simulink model "spaceShuttleOriginal"  (R2017b)
settings: Solver=FixedStepAuto  StartTime=0.0  StopTime=300  FixedStep=0.08  RelTol=1e-3
undefined symbols (not defined in the file or in its folder): ATTITUDE_ESTIMATE, ATTITUDE_INCREMENT, AUTO_MANUAL_SWITCH, BYPASS, COUNTER, CURRENT_ATTITUDE, DESIRED_ATTITUDE, DESIRED_RATE, INIT_AUTO_MANEUVER, INIT_JET_SELECT, INIT_STATE_ERROR, MANEUVER_HOLD_SW, PRIMARY_JET_COMMAND, RATE_ESTIMATE, UNDESIRED_ACCELERATION_ESTIMATE, VERNIER_JET_COMMAND
libraries: sharedtransform x5, aerolibutil x4, realtime_pacer_lib x1
(part 2 of 3)

== system spaceShuttleOriginal/State Error/Coordinate 2 ==
  In1 : Inport
  Bus Selector : BusSelector  OutputSignals=INIT_STATE_ERROR
  INIT STATE ERROR = OFF : Subsystem  TreatAsAtomicUnit=on
  INIT STATE ERROR = ON : Subsystem  TreatAsAtomicUnit=on
  If : If  IfExpression=u1 == 1
  Merge : Merge
  Selector : Selector  InputPortWidth=3  IndexOptions=Index vector (dialog)  Indices=[2]  OutputSizes=1
  y : Outport
  wires:
  Merge/1 -> y/1
  In1/1 -> INIT STATE ERROR = OFF/1(In1), INIT STATE ERROR = ON/1(In1), Bus Selector/1
  If/2 -> INIT STATE ERROR = OFF/Action
  INIT STATE ERROR = ON/1(y) -> Merge/1
  If/1 -> INIT STATE ERROR = ON/Action
  Selector/1 -> If/1
  INIT STATE ERROR = OFF/1(y1) -> Merge/2
  Bus Selector/1 -> Selector/1  "<INIT_STATE_ERROR>"

== system spaceShuttleOriginal/State Error/Coordinate 3 ==
  In2 : Inport
  Bus Selector : BusSelector  OutputSignals=INIT_STATE_ERROR
  INIT STATE ERROR = OFF : Subsystem  TreatAsAtomicUnit=on
  INIT STATE ERROR = ON : Subsystem  TreatAsAtomicUnit=on
  If : If  IfExpression=u1 == 1
  Merge : Merge
  Selector : Selector  InputPortWidth=3  IndexOptions=Index vector (dialog)  Indices=[3]  OutputSizes=1
  y1 : Outport
  wires:
  Merge/1 -> y1/1
  In2/1 -> INIT STATE ERROR = OFF/1(In1), INIT STATE ERROR = ON/1(In1), Bus Selector/1
  If/2 -> INIT STATE ERROR = OFF/Action
  INIT STATE ERROR = ON/1(y) -> Merge/1
  If/1 -> INIT STATE ERROR = ON/Action
  Selector/1 -> If/1
  INIT STATE ERROR = OFF/1(y1) -> Merge/2
  Bus Selector/1 -> Selector/1  "<INIT_STATE_ERROR>"

== system spaceShuttleOriginal/Update Auto Manual Switch/IF RHC ==
  In1 : Inport
  Action Port : ActionPort  ActionType=then
  Bus Assignment : BusAssignment  AssignedSignals=AUTO_MANUAL_SWITCH
  Constant1 : Constant  Value=0
  Data Store Read : DataStoreRead  DataStoreName=AUTO_MANUAL_SWITCH  DataStoreElements=AUTO_MANUAL_SWITCH(1)
  Data Store Write1 : DataStoreWrite  DataStoreName=AUTO_MANUAL_SWITCH
  Mux : Mux  Inputs=2
  x : Outport
  wires:
  Mux/1 -> Bus Assignment/2, Data Store Write1/1
  Data Store Read/1 -> Mux/2
  Constant1/1 -> Mux/1
  In1/1 -> Bus Assignment/1
  Bus Assignment/1 -> x/1

== system spaceShuttleOriginal/Update Auto Manual Switch/NO RHC ==
  In1 : Inport
  Action Port : ActionPort  ActionType=else
  Bus Assignment : BusAssignment  AssignedSignals=AUTO_MANUAL_SWITCH
  Constant1 : Constant
  Data Store Read : DataStoreRead  DataStoreName=AUTO_MANUAL_SWITCH  DataStoreElements=AUTO_MANUAL_SWITCH(1)
  Data Store Write1 : DataStoreWrite  DataStoreName=AUTO_MANUAL_SWITCH
  Mux : Mux  Inputs=2
  x1 : Outport
  wires:
  Mux/1 -> Bus Assignment/2, Data Store Write1/1
  Constant1/1 -> Mux/1
  Data Store Read/1 -> Mux/2
  Bus Assignment/1 -> x1/1
  In1/1 -> Bus Assignment/1

== system spaceShuttleOriginal/VISUALIZATION AND COMMANDS/Knob1 ==

== system spaceShuttleOriginal/VISUALIZATION AND COMMANDS/Knob2 ==

== system spaceShuttleOriginal/VISUALIZATION AND COMMANDS/Knob3 ==

== system spaceShuttleOriginal/VISUALIZATION AND COMMANDS/Knob4 ==

== system spaceShuttleOriginal/VISUALIZATION AND COMMANDS/Knob5 ==

== system spaceShuttleOriginal/VISUALIZATION AND COMMANDS/Lamp ==

== system spaceShuttleOriginal/VISUALIZATION AND COMMANDS/Lamp1 ==

== system spaceShuttleOriginal/VISUALIZATION AND COMMANDS/Lamp10 ==

== system spaceShuttleOriginal/VISUALIZATION AND COMMANDS/Lamp2 ==

== system spaceShuttleOriginal/VISUALIZATION AND COMMANDS/Lamp3 ==

== system spaceShuttleOriginal/VISUALIZATION AND COMMANDS/Lamp4 ==

== system spaceShuttleOriginal/VISUALIZATION AND COMMANDS/Lamp5 ==

== system spaceShuttleOriginal/VISUALIZATION AND COMMANDS/Lamp6 ==

== system spaceShuttleOriginal/VISUALIZATION AND COMMANDS/Lamp7 ==

== system spaceShuttleOriginal/VISUALIZATION AND COMMANDS/Lamp8 ==

== system spaceShuttleOriginal/VISUALIZATION AND COMMANDS/Lamp9 ==

== system spaceShuttleOriginal/VISUALIZATION AND COMMANDS/Rotary Switch ==

== system spaceShuttleOriginal/VISUALIZATION AND COMMANDS/Rotary Switch1 ==

== system spaceShuttleOriginal/VISUALIZATION AND COMMANDS/Rotary Switch2 ==

== system spaceShuttleOriginal/VISUALIZATION AND COMMANDS/Toggle Switch ==

== system spaceShuttleOriginal/VISUALIZATION AND COMMANDS/Toggle Switch1 ==

== system spaceShuttleOriginal/VISUALIZATION AND COMMANDS/Toggle Switch2 ==

== system spaceShuttleOriginal/VISUALIZATION AND COMMANDS/Toggle Switch3 ==

== system spaceShuttleOriginal/Attitude Processing/SECOND_PASS == 1/ATTITUDE PROCESSOR ==
  R_I_B : Inport
  R_I_B_PREVIOUS : Inport  Port=2
  Direction Cosine Matrix to Quaternions : sharedtransform/Direction Cosine Matrix  to Quaternions
      settings: SourceProductName=Aerospace Blockset  SourceProductBaseCode=AE
  Direction Cosine Matrix to Quaternions1 : sharedtransform/Direction Cosine Matrix  to Quaternions
      settings: SourceProductName=Aerospace Blockset  SourceProductBaseCode=AE
  Direction Cosine Matrix to Quaternions2 : sharedtransform/Direction Cosine Matrix  to Quaternions
      settings: SourceProductName=Aerospace Blockset  SourceProductBaseCode=AE
  Display1 : Display
  Display2 : Display
  Display3 : Display
  MATLAB Function2 : MATLAB Function  TreatAsAtomicUnit=on
  MATLAB Function3 : MATLAB Function  TreatAsAtomicUnit=on
  Quaternion Conjugate : aerolibutil/Quaternion Conjugate
      settings: SourceProductName=Aerospace Blockset  SourceProductBaseCode=AE
  Quaternion Multiplication : aerolibutil/Quaternion Multiplication
  Scope : Scope
  Scope1 : Scope
  To Workspace : ToWorkspace  VariableName=test1  SaveFormat=Timeseries  SampleTime=-1
  CURRENT ATTITUDE : Outport
  ATTITUDE INCREMENT : Outport  Port=2
  wires:
  R_I_B/1 -> Direction Cosine Matrix to Quaternions1/1, MATLAB Function3/1(u), Direction Cosine Matrix to Quaternions/1
  Direction Cosine Matrix to Quaternions/1 -> To Workspace/1, Scope/1, Display1/1, CURRENT ATTITUDE/1
  R_I_B_PREVIOUS/1 -> Direction Cosine Matrix to Quaternions2/1
  MATLAB Function2/1(x) -> Scope1/1, Display3/1, ATTITUDE INCREMENT/1
  MATLAB Function3/1(x) -> Display2/1
  Direction Cosine Matrix to Quaternions2/1 -> Quaternion Conjugate/1
  Direction Cosine Matrix to Quaternions1/1 -> Quaternion Multiplication/1
  Quaternion Conjugate/1 -> Quaternion Multiplication/2
  Quaternion Multiplication/1 -> MATLAB Function2/1(u)

== system spaceShuttleOriginal/Attitude Processing/SECOND_PASS == 1/State Estimator Part I ==
  CURRENT_ATTITUDE : Inport
  Derivative1 : Derivative
  Derivative2 : Derivative
  MATLAB Function2 : MATLAB Function  TreatAsAtomicUnit=on
  ATTITUDE_ESTIMATE : Outport
  RATE_ESTIMATE : Outport  Port=2
  UNDESIRED_ACCELERATION_ESTIMATE : Outport  Port=3
  wires:
  Derivative1/1 -> Derivative2/1, RATE_ESTIMATE/1
  Derivative2/1 -> UNDESIRED_ACCELERATION_ESTIMATE/1
  CURRENT_ATTITUDE/1 -> MATLAB Function2/1(u)
  MATLAB Function2/1(x) -> ATTITUDE_ESTIMATE/1, Derivative1/1

== system spaceShuttleOriginal/Auto // Manual Maneuver/IF MANUAL/MANUAL MANEUVER MODULE ==
  In1 : Inport
  Affect Coordinate 1 : Subsystem
  Affect Coordinate 2 : Subsystem
  Affect Coordinate 3 : Subsystem
  Out1 : Outport
  wires:
  In1/1 -> Affect Coordinate 1/1(In1)
  Affect Coordinate 1/1(Out1) -> Affect Coordinate 2/1(In1)
  Affect Coordinate 2/1(Out1) -> Affect Coordinate 3/1(In1)
  Affect Coordinate 3/1(Out1) -> Out1/1

== system spaceShuttleOriginal/Auto // Manual Maneuver/If AUTO/COUNTER ~=0 ==
  In1 : Inport
  Action Port : ActionPort  ActionType=else
  Out1 : Outport
  wires:
  In1/1 -> Out1/1

== system spaceShuttleOriginal/Auto // Manual Maneuver/If AUTO/IF COUNTER=0 ==
  In2 : Inport
  Action Port : ActionPort  ActionType=then
  AUTO MANEUVER MODULE : Subsystem
  Bus Assignment : BusAssignment  AssignedSignals=COUNTER
  Constant2 : Constant  Value=12
  Data Store Write1 : DataStoreWrite  DataStoreName=COUNTER
  Out1 : Outport
  wires:
  Constant2/1 -> Bus Assignment/2, Data Store Write1/1
  AUTO MANEUVER MODULE/1(Out1) -> Out1/1
  Bus Assignment/1 -> AUTO MANEUVER MODULE/1(In1)
  In2/1 -> Bus Assignment/1

== system spaceShuttleOriginal/Auto // Manual Maneuver/If AUTO/IF OLD=AUTO ==
  In1 : Inport
  Action Port : ActionPort  ActionType=else
  Out1 : Outport
  wires:
  In1/1 -> Out1/1

== system spaceShuttleOriginal/Auto // Manual Maneuver/If AUTO/IF OLD=MANUAL ==
  In1 : Inport
  Action Port : ActionPort  ActionType=then
  Bus Assignment : BusAssignment  AssignedSignals=BYPASS,INIT_AUTO_MANEUVER,COUNTER
  Constant{1..4} (4 alike) : Constant  Value=0
  Constant5 : Constant
  Data Store Write : DataStoreWrite  DataStoreName=BYPASS
  Data Store Write1 : DataStoreWrite  DataStoreName=COUNTER
  Data Store Write2 : DataStoreWrite  DataStoreName=INIT_AUTO_MANEUVER
  Mux : Mux  Inputs=3
  Out1 : Outport
  wires:
  Constant2/1 -> Bus Assignment/4, Data Store Write1/1
  Constant1/1 -> Mux/1
  Constant3/1 -> Mux/2
  Constant4/1 -> Mux/3
  Mux/1 -> Bus Assignment/2, Data Store Write/1
  Constant5/1 -> Bus Assignment/3, Data Store Write2/1
  In1/1 -> Bus Assignment/1
  Bus Assignment/1 -> Out1/1

== system spaceShuttleOriginal/First Pass/If First Pass/AUTO ==
  In2 : Inport
  Action Port : ActionPort  ActionType=else
  Bus Assignment1 : BusAssignment  AssignedSignals=INIT_STATE_ERROR
  Data Store Read : DataStoreRead  DataStoreName=INIT_STATE_ERROR
  x1 : Outport
  wires:
  Data Store Read/1 -> Bus Assignment1/2
  In2/1 -> Bus Assignment1/1
  Bus Assignment1/1 -> x1/1

== system spaceShuttleOriginal/First Pass/If First Pass/MANUAL ==
  In1 : Inport
  Action Port : ActionPort  ActionType=then
  Bus Assignment : BusAssignment  AssignedSignals=INIT_STATE_ERROR
  Constant2 : Constant  Value=[1;1;1]
  Data Store Write1 : DataStoreWrite  DataStoreName=INIT_STATE_ERROR
  x : Outport
  wires:
  In1/1 -> Bus Assignment/1
  Bus Assignment/1 -> x/1
  Constant2/1 -> Data Store Write1/1, Bus Assignment/2

== system spaceShuttleOriginal/State Error/Coordinate 1/INIT STATE ERROR = OFF ==
  In1 : Inport
  Action Port : ActionPort  ActionType=else
  y1 : Outport
  wires:
  In1/1 -> y1/1

== system spaceShuttleOriginal/State Error/Coordinate 1/INIT STATE ERROR = ON ==
  In1 : Inport
  Action Port : ActionPort  ActionType=then
  Bus Assignment : BusAssignment  AssignedSignals=DESIRED_ATTITUDE
  Bus Assignment1 : BusAssignment  AssignedSignals=INIT_STATE_ERROR
  Bus Selector : BusSelector  OutputSignals=DESIRED_ATTITUDE,ATTITUDE_ESTIMATE
  Bus Selector1 : BusSelector  OutputSignals=INIT_STATE_ERROR
  Constant : Constant  Value=0
  Data Store Write1 : DataStoreWrite  DataStoreName=INIT_STATE_ERROR
  Data Store Write3 : DataStoreWrite  DataStoreName=DESIRED_ATTITUDE
  Demux : Demux  Outputs=3
  Demux1 : Demux  Outputs=3
  Mux : Mux  Inputs=3
  Mux1 : Mux  Inputs=3
  Selector : Selector  InputPortWidth=3  IndexOptions=Index vector (dialog)  Indices=[1]  OutputSizes=1
  Terminator : Terminator
  Terminator1 : Terminator
  y : Outport
  wires:
  In1/1 -> Bus Assignment/1, Bus Selector/1
  Bus Selector/1 -> Demux/1  "<DESIRED_ATTITUDE>"
  Bus Selector/2 -> Selector/1  "<ATTITUDE_ESTIMATE>"
  Selector/1 -> Mux/1
  Demux/2 -> Mux/2
  Demux/3 -> Mux/3
  Mux/1 -> Data Store Write3/1, Bus Assignment/2
  Bus Selector1/1 -> Demux1/1  "<INIT_STATE_ERROR>"
  Demux1/3 -> Mux1/3
  Bus Assignment1/1 -> y/1
  Mux1/1 -> Bus Assignment1/2, Data Store Write1/1
  Bus Assignment/1 -> Bus Assignment1/1, Bus Selector1/1
  Demux1/2 -> Mux1/2
  Constant/1 -> Mux1/1
  Demux/1 -> Terminator/1
  Demux1/1 -> Terminator1/1

== system spaceShuttleOriginal/State Error/Coordinate 2/INIT STATE ERROR = OFF ==
  In1 : Inport
  Action Port : ActionPort  ActionType=else
  y1 : Outport
  wires:
  In1/1 -> y1/1

== system spaceShuttleOriginal/State Error/Coordinate 2/INIT STATE ERROR = ON ==
  In1 : Inport
  Action Port : ActionPort  ActionType=then
  Bus Assignment : BusAssignment  AssignedSignals=DESIRED_ATTITUDE
  Bus Assignment1 : BusAssignment  AssignedSignals=INIT_STATE_ERROR
  Bus Selector : BusSelector  OutputSignals=DESIRED_ATTITUDE,ATTITUDE_ESTIMATE
  Bus Selector1 : BusSelector  OutputSignals=INIT_STATE_ERROR
  Constant : Constant  Value=0
  Data Store Write1 : DataStoreWrite  DataStoreName=INIT_STATE_ERROR
  Data Store Write3 : DataStoreWrite  DataStoreName=DESIRED_ATTITUDE
  Demux : Demux  Outputs=3
  Demux1 : Demux  Outputs=3
  Mux : Mux  Inputs=3
  Mux1 : Mux  Inputs=3
  Selector : Selector  InputPortWidth=3  IndexOptions=Index vector (dialog)  Indices=[2]  OutputSizes=1
  Terminator : Terminator
  Terminator1 : Terminator
  y : Outport
  wires:
  In1/1 -> Bus Assignment/1, Bus Selector/1
  Bus Selector/1 -> Demux/1  "<DESIRED_ATTITUDE>"
  Bus Selector/2 -> Selector/1  "<ATTITUDE_ESTIMATE>"
  Mux/1 -> Data Store Write3/1, Bus Assignment/2
  Bus Selector1/1 -> Demux1/1  "<INIT_STATE_ERROR>"
  Bus Assignment1/1 -> y/1
  Mux1/1 -> Bus Assignment1/2, Data Store Write1/1
  Bus Assignment/1 -> Bus Assignment1/1, Bus Selector1/1
  Selector/1 -> Mux/2
  Demux/3 -> Mux/3
  Demux/1 -> Mux/1
  Constant/1 -> Mux1/2
  Demux1/1 -> Mux1/1
  Demux1/3 -> Mux1/3
  Demux/2 -> Terminator/1
  Demux1/2 -> Terminator1/1

== system spaceShuttleOriginal/State Error/Coordinate 3/INIT STATE ERROR = OFF ==
  In1 : Inport
  Action Port : ActionPort  ActionType=else
  y1 : Outport
  wires:
  In1/1 -> y1/1

== system spaceShuttleOriginal/State Error/Coordinate 3/INIT STATE ERROR = ON ==
  In1 : Inport
  Action Port : ActionPort  ActionType=then
  Bus Assignment : BusAssignment  AssignedSignals=DESIRED_ATTITUDE
  Bus Assignment1 : BusAssignment  AssignedSignals=INIT_STATE_ERROR
  Bus Selector : BusSelector  OutputSignals=DESIRED_ATTITUDE,ATTITUDE_ESTIMATE
  Bus Selector1 : BusSelector  OutputSignals=INIT_STATE_ERROR
  Constant : Constant  Value=0
  Data Store Write1 : DataStoreWrite  DataStoreName=INIT_STATE_ERROR
  Data Store Write3 : DataStoreWrite  DataStoreName=DESIRED_ATTITUDE
  Demux : Demux  Outputs=3
  Demux1 : Demux  Outputs=3
  Mux : Mux  Inputs=3
  Mux1 : Mux  Inputs=3
  Selector : Selector  InputPortWidth=3  IndexOptions=Index vector (dialog)  Indices=[3]  OutputSizes=1
  Terminator : Terminator
  Terminator1 : Terminator
  y : Outport
  wires:
  In1/1 -> Bus Assignment/1, Bus Selector/1
  Bus Selector/1 -> Demux/1  "<DESIRED_ATTITUDE>"
  Bus Selector/2 -> Selector/1  "<ATTITUDE_ESTIMATE>"
  Mux/1 -> Data Store Write3/1, Bus Assignment/2
  Bus Selector1/1 -> Demux1/1  "<INIT_STATE_ERROR>"
  Bus Assignment1/1 -> y/1
  Mux1/1 -> Bus Assignment1/2, Data Store Write1/1
  Bus Assignment/1 -> Bus Assignment1/1, Bus Selector1/1
  Selector/1 -> Mux/3
  Demux/2 -> Mux/2
  Demux/1 -> Mux/1
  Constant/1 -> Mux1/3
  Demux1/2 -> Mux1/2
  Demux1/1 -> Mux1/1
  Demux/3 -> Terminator/1
  Demux1/3 -> Terminator1/1

== system spaceShuttleOriginal/Auto // Manual Maneuver/IF MANUAL/MANUAL MANEUVER MODULE/Affect Coordinate 1 ==
  In1 : Inport
  Bus Selector : BusSelector  OutputSignals=USER_INPUTS.CLOSED_LOOP
  CLOSED LOOP = OFF : Subsystem  TreatAsAtomicUnit=on
  CLOSED LOOP = ON : Subsystem  TreatAsAtomicUnit=on
  If : If  IfExpression=u1 == 1
  Merge : Merge
  Selector : Selector  InputPortWidth=3  IndexOptions=Index vector (dialog)  Indices=[1]  OutputSizes=1
  Out1 : Outport
  wires:
  In1/1 -> CLOSED LOOP = ON/1(x), CLOSED LOOP = OFF/1(x), Bus Selector/1
  Bus Selector/1 -> Selector/1  "<CLOSED_LOOP>"
  Merge/1 -> Out1/1
  CLOSED LOOP = OFF/1(y) -> Merge/2
  Selector/1 -> If/1
  If/2 -> CLOSED LOOP = OFF/Action
  If/1 -> CLOSED LOOP = ON/Action
  CLOSED LOOP = ON/1(Out2) -> Merge/1

== system spaceShuttleOriginal/Auto // Manual Maneuver/IF MANUAL/MANUAL MANEUVER MODULE/Affect Coordinate 2 ==
  In1 : Inport
  Bus Selector : BusSelector  OutputSignals=USER_INPUTS.CLOSED_LOOP
  CLOSED LOOP = OFF : Subsystem  TreatAsAtomicUnit=on
  CLOSED LOOP = ON : Subsystem  TreatAsAtomicUnit=on
  If : If  IfExpression=u1 == 1
  Merge : Merge
  Selector : Selector  InputPortWidth=3  IndexOptions=Index vector (dialog)  Indices=[2]  OutputSizes=1
  Out1 : Outport
  wires:
  In1/1 -> CLOSED LOOP = OFF/1(x), CLOSED LOOP = ON/1(x), Bus Selector/1
  Bus Selector/1 -> Selector/1  "<CLOSED_LOOP>"
  Merge/1 -> Out1/1
  CLOSED LOOP = OFF/1(y) -> Merge/2
  Selector/1 -> If/1
  If/2 -> CLOSED LOOP = OFF/Action
  If/1 -> CLOSED LOOP = ON/Action
  CLOSED LOOP = ON/1(Out1) -> Merge/1

== system spaceShuttleOriginal/Auto // Manual Maneuver/IF MANUAL/MANUAL MANEUVER MODULE/Affect Coordinate 3 ==
  In1 : Inport
  Bus Selector : BusSelector  OutputSignals=USER_INPUTS.CLOSED_LOOP
  CLOSED LOOP = OFF : Subsystem  TreatAsAtomicUnit=on
  CLOSED LOOP = ON : Subsystem  TreatAsAtomicUnit=on
  If : If  IfExpression=u1 == 1
  Merge : Merge
  Selector : Selector  InputPortWidth=3  IndexOptions=Index vector (dialog)  Indices=[3]  OutputSizes=1
  Out1 : Outport
  wires:
  In1/1 -> CLOSED LOOP = ON/1(x), CLOSED LOOP = OFF/1(x), Bus Selector/1
  Bus Selector/1 -> Selector/1  "<CLOSED_LOOP>"
  Merge/1 -> Out1/1
  CLOSED LOOP = OFF/1(y) -> Merge/2
  Selector/1 -> If/1
  If/2 -> CLOSED LOOP = OFF/Action
  If/1 -> CLOSED LOOP = ON/Action
  CLOSED LOOP = ON/1(Out1) -> Merge/1

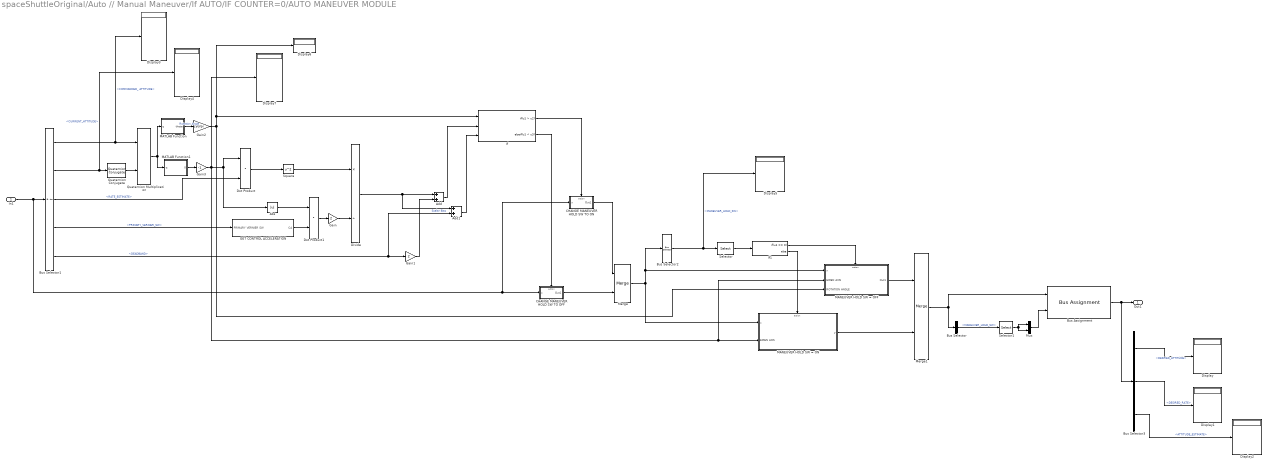
== system spaceShuttleOriginal/Auto // Manual Maneuver/If AUTO/IF COUNTER=0/AUTO MANEUVER MODULE ==
  In1 : Inport
  Abs : Abs
  Add : Sum
  Add1 : Sum
  Bus Assignment : BusAssignment  AssignedSignals=MANEUVER_HOLD_SW
  Bus Selector : BusSelector  OutputSignals=MANEUVER_HOLD_SW
  Bus Selector1 : BusSelector  OutputSignals=USER_INPUTS.COMMANDED_ ATTITUDE,CURRENT_ATTITUDE,RATE_ESTIMATE,USER_INPUTS.PRIMARY_VERNIER_SW,USER_INPUTS.DEADBAND
  Bus Selector2 : BusSelector  OutputSignals=MANEUVER_HOLD_SW
  Bus Selector3 : BusSelector  OutputSignals=DESIRED_ATTITUDE,DESIRED_RATE,ATTITUDE_ESTIMATE
  CHANGE MANEUVER HOLD SW TO OFF : Subsystem  TreatAsAtomicUnit=on
  CHANGE MANEUVER HOLD SW TO ON : Subsystem  TreatAsAtomicUnit=on
  Display{,1..7} (8 alike) : Display
  Divide : Product  Inputs=*/
  Dot Product : DotProduct  InputSameDT=on  OutDataTypeStr=Inherit: Inherit via internal rule
  Dot Product1 : DotProduct  InputSameDT=on  OutDataTypeStr=Inherit: Inherit via internal rule
  GET CONTROL ACCELERATION : Subsystem
  Gain : Gain  Gain=2
  Gain1 : Gain  Gain=2
  Gain2 : Gain  Gain=180/pi
  Gain3 : Gain  Gain=-1
  If : If  NumInputs=3  IfExpression=u1 > u2  ElseIfExpressions=u1 < u3  ShowElse=off
  If1 : If  IfExpression=u1 == 0
  MANEUVER HOLD SW = OFF : Subsystem  TreatAsAtomicUnit=on
  MANEUVER HOLD SW = ON : Subsystem  TreatAsAtomicUnit=on
  MATLAB Function : MATLAB Function  TreatAsAtomicUnit=on
  MATLAB Function1 : MATLAB Function  TreatAsAtomicUnit=on
  Merge : Merge
  Merge1 : Merge
  Mux : Mux  Inputs=2
  Quaternion Conjugate : aerolibutil/Quaternion Conjugate
      settings: SourceProductName=Aerospace Blockset  SourceProductBaseCode=AE
  Quaternion Multiplication : aerolibutil/Quaternion Multiplication
  Selector : Selector  InputPortWidth=2  IndexOptions=Index vector (dialog)  Indices=[1]  OutputSizes=1
  Selector1 : Selector  InputPortWidth=2  IndexOptions=Index vector (dialog)  Indices=[1]  OutputSizes=1
  Square : Math  Operator=square  RndMeth=Zero  SaturateOnIntegerOverflow=on
  Out1 : Outport
  wires:
  MANEUVER HOLD SW = ON/1(y) -> Merge1/2
  Gain/1 -> Divide/2
  Divide/1 -> Add1/1, Add/1  "Scalar Bias"
  Merge/1 -> MANEUVER HOLD SW = ON/1(x), Bus Selector2/1, MANEUVER HOLD SW = OFF/1(x)
  If1/1 -> MANEUVER HOLD SW = OFF/Action
  CHANGE MANEUVER HOLD SW TO OFF/1(Out1) -> Merge/2
  MANEUVER HOLD SW = OFF/1(Out1) -> Merge1/1
  Selector/1 -> If1/1
  MATLAB Function1/1(U) -> Gain3/1
  Gain1/1 -> Add/2
  Add/1 -> If/2
  In1/1 -> Bus Selector1/1, CHANGE MANEUVER HOLD SW TO OFF/1(x), CHANGE MANEUVER HOLD SW TO ON/1(x)
  GET CONTROL ACCELERATION/1(CA) -> Dot Product1/2
  If/1 -> CHANGE MANEUVER HOLD SW TO ON/Action
  Square/1 -> Divide/1
  Dot Product1/1 -> Gain/1
  Add1/1 -> If/3
  MATLAB Function/1(theta) -> Gain2/1  "Rotation Angle"
  If/2 -> CHANGE MANEUVER HOLD SW TO OFF/Action
  Abs/1 -> Dot Product1/1
  Quaternion Multiplication/1 -> MATLAB Function/1(q), MATLAB Function1/1(q)
  If1/2 -> MANEUVER HOLD SW = ON/Action
  Quaternion Conjugate/1 -> Quaternion Multiplication/2
  Dot Product/1 -> Square/1
  CHANGE MANEUVER HOLD SW TO ON/1(Out1) -> Merge/1
  Bus Selector2/1 -> Display5/1, Selector/1  "<MANEUVER_HOLD_SW>"
  Merge1/1 -> Bus Selector/1, Bus Assignment/1
  Bus Selector/1 -> Selector1/1  "<MANEUVER_HOLD_SW>"
  Mux/1 -> Bus Assignment/2
  Selector1/1 -> Mux/1, Mux/2
  Bus Selector3/2 -> Display1/1  "<DESIRED_RATE>"
  Bus Selector3/1 -> Display/1  "<DESIRED_ATTITUDE>"
  Bus Assignment/1 -> Bus Selector3/1, Out1/1
  Bus Selector3/3 -> Display2/1  "<ATTITUDE_ESTIMATE>"
  Gain2/1 -> MANEUVER HOLD SW = OFF/3(ROTATION ANGLE), Display6/1, If/1
  Gain3/1 -> Display7/1, MANEUVER HOLD SW = OFF/2(EIGEN AXIS), MANEUVER HOLD SW = ON/2(EIGEN AXIS), Abs/1, Dot Product/1
  Bus Selector1/2 -> Quaternion Conjugate/1, Display4/1  "<CURRENT_ATTITUDE>"
  Bus Selector1/3 -> Dot Product/2  "<RATE_ESTIMATE>"
  Bus Selector1/4 -> GET CONTROL ACCELERATION/1(PRIMARY VERNIER SW)  "<PRIMARY_VERNIER_SW>"
  Bus Selector1/5 -> Add1/2, Gain1/1  "<DEADBAND>"
  Bus Selector1/1 -> Quaternion Multiplication/1, Display3/1  "<COMMANDED_ ATTITUDE>"

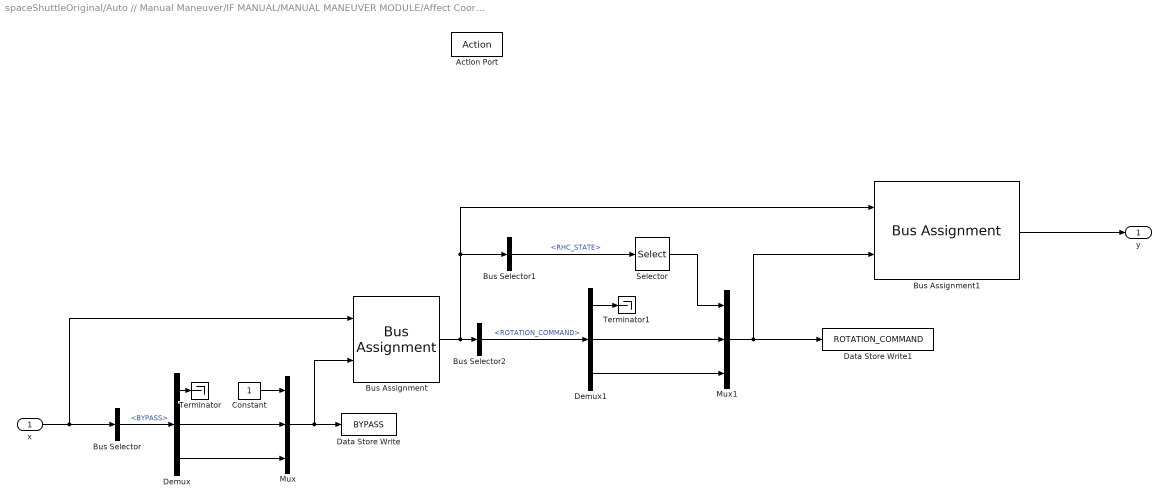
== system spaceShuttleOriginal/Auto // Manual Maneuver/IF MANUAL/MANUAL MANEUVER MODULE/Affect Coordinate 1/CLOSED LOOP = OFF ==
  x : Inport
  Action Port : ActionPort  ActionType=else
  Bus Assignment : BusAssignment  AssignedSignals=BYPASS
  Bus Assignment1 : BusAssignment  AssignedSignals=ROTATION_COMMAND
  Bus Selector : BusSelector  OutputSignals=BYPASS
  Bus Selector1 : BusSelector  OutputSignals=USER_INPUTS.RHC_STATE
  Bus Selector2 : BusSelector  OutputSignals=ROTATION_COMMAND
  Constant : Constant
  Data Store Write : DataStoreWrite  DataStoreName=BYPASS
  Data Store Write1 : DataStoreWrite  DataStoreName=ROTATION_COMMAND
  Demux : Demux  Outputs=3
  Demux1 : Demux  Outputs=3
  Mux : Mux  Inputs=3
  Mux1 : Mux  Inputs=3
  Selector : Selector  InputPortWidth=3  IndexOptions=Index vector (dialog)  Indices=[1]  OutputSizes=1
  Terminator : Terminator
  Terminator1 : Terminator
  y : Outport
  wires:
  x/1 -> Bus Assignment/1, Bus Selector/1
  Bus Selector/1 -> Demux/1  "<BYPASS>"
  Demux/3 -> Mux/3
  Demux/2 -> Mux/2
  Constant/1 -> Mux/1
  Mux/1 -> Data Store Write/1, Bus Assignment/2
  Demux/1 -> Terminator/1
  Bus Assignment/1 -> Bus Assignment1/1, Bus Selector1/1, Bus Selector2/1
  Mux1/1 -> Data Store Write1/1, Bus Assignment1/2
  Demux1/2 -> Mux1/2
  Demux1/3 -> Mux1/3
  Bus Selector2/1 -> Demux1/1  "<ROTATION_COMMAND>"
  Demux1/1 -> Terminator1/1
  Bus Selector1/1 -> Selector/1  "<RHC_STATE>"
  Selector/1 -> Mux1/1
  Bus Assignment1/1 -> y/1

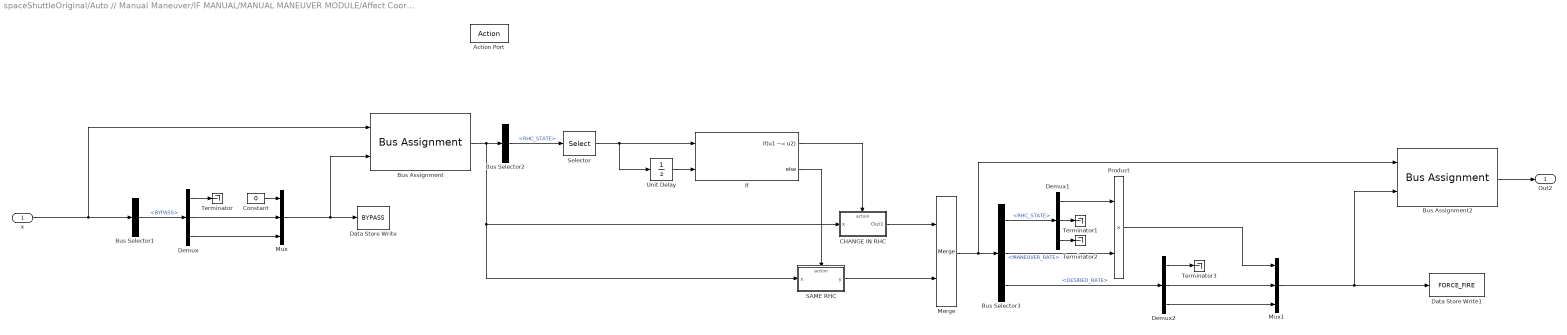
== system spaceShuttleOriginal/Auto // Manual Maneuver/IF MANUAL/MANUAL MANEUVER MODULE/Affect Coordinate 1/CLOSED LOOP = ON ==
  x : Inport
  Action Port : ActionPort  ActionType=then
  Bus Assignment : BusAssignment  AssignedSignals=BYPASS
  Bus Assignment2 : BusAssignment  AssignedSignals=FORCE_FIRE
  Bus Selector1 : BusSelector  OutputSignals=BYPASS
  Bus Selector2 : BusSelector  OutputSignals=USER_INPUTS.RHC_STATE
  Bus Selector3 : BusSelector  OutputSignals=USER_INPUTS.RHC_STATE,USER_INPUTS.MANEUVER_RATE,DESIRED_RATE
  CHANGE IN RHC : Subsystem  TreatAsAtomicUnit=on
  Constant : Constant  Value=0
  Data Store Write : DataStoreWrite  DataStoreName=BYPASS
  Data Store Write1 : DataStoreWrite  DataStoreName=FORCE_FIRE
  Demux : Demux  Outputs=3
  Demux1 : Demux  Outputs=3
  Demux2 : Demux  Outputs=3
  If : If  NumInputs=2  IfExpression=u1 ~= u2
  Merge : Merge
  Mux : Mux  Inputs=3
  Mux1 : Mux  Inputs=3
  Product : Product
  SAME RHC : Subsystem  TreatAsAtomicUnit=on
  Selector : Selector  InputPortWidth=3  IndexOptions=Index vector (dialog)  Indices=[1]  OutputSizes=1
  Terminator{,1..3} (4 alike) : Terminator
  Unit Delay : UnitDelay  SampleTime=-1
  Out2 : Outport
  wires:
  x/1 -> Bus Assignment/1, Bus Selector1/1
  Bus Selector1/1 -> Demux/1  "<BYPASS>"
  Constant/1 -> Mux/1
  Demux/2 -> Mux/2
  Demux/3 -> Mux/3
  Mux/1 -> Data Store Write/1, Bus Assignment/2
  Bus Assignment/1 -> CHANGE IN RHC/1(x), SAME RHC/1(x), Bus Selector2/1
  Bus Selector2/1 -> Selector/1  "<RHC_STATE>"
  Selector/1 -> Unit Delay/1, If/1
  Unit Delay/1 -> If/2
  SAME RHC/1(y) -> Merge/2
  If/2 -> SAME RHC/Action
  If/1 -> CHANGE IN RHC/Action
  CHANGE IN RHC/1(Out1) -> Merge/1
  Merge/1 -> Bus Assignment2/1, Bus Selector3/1
  Bus Selector3/1 -> Demux1/1  "<RHC_STATE>"
  Bus Assignment2/1 -> Out2/1
  Demux1/1 -> Product/1
  Bus Selector3/2 -> Product/2  "<MANEUVER_RATE>"
  Product/1 -> Mux1/1
  Bus Selector3/3 -> Demux2/1  "<DESIRED_RATE>"
  Demux2/3 -> Mux1/3
  Demux2/2 -> Mux1/2
  Mux1/1 -> Bus Assignment2/2, Data Store Write1/1
  Demux/1 -> Terminator/1
  Demux1/2 -> Terminator1/1
  Demux1/3 -> Terminator2/1
  Demux2/1 -> Terminator3/1

== system spaceShuttleOriginal/Auto // Manual Maneuver/IF MANUAL/MANUAL MANEUVER MODULE/Affect Coordinate 2/CLOSED LOOP = OFF ==
  x : Inport
  Action Port : ActionPort  ActionType=else
  Bus Assignment : BusAssignment  AssignedSignals=BYPASS
  Bus Assignment1 : BusAssignment  AssignedSignals=ROTATION_COMMAND
  Bus Selector : BusSelector  OutputSignals=BYPASS
  Bus Selector1 : BusSelector  OutputSignals=USER_INPUTS.RHC_STATE
  Bus Selector2 : BusSelector  OutputSignals=ROTATION_COMMAND
  Constant : Constant
  Data Store Write : DataStoreWrite  DataStoreName=BYPASS
  Data Store Write1 : DataStoreWrite  DataStoreName=ROTATION_COMMAND
  Demux : Demux  Outputs=3
  Demux1 : Demux  Outputs=3
  Mux : Mux  Inputs=3
  Mux1 : Mux  Inputs=3
  Selector : Selector  InputPortWidth=3  IndexOptions=Index vector (dialog)  Indices=[2]  OutputSizes=1
  Terminator : Terminator
  Terminator1 : Terminator
  y : Outport
  wires:
  x/1 -> Bus Assignment/1, Bus Selector/1
  Bus Selector/1 -> Demux/1  "<BYPASS>"
  Mux/1 -> Data Store Write/1, Bus Assignment/2
  Bus Assignment/1 -> Bus Assignment1/1, Bus Selector1/1, Bus Selector2/1
  Mux1/1 -> Data Store Write1/1, Bus Assignment1/2
  Bus Selector2/1 -> Demux1/1  "<ROTATION_COMMAND>"
  Bus Selector1/1 -> Selector/1  "<RHC_STATE>"
  Bus Assignment1/1 -> y/1
  Demux1/2 -> Terminator1/1
  Selector/1 -> Mux1/2
  Demux1/1 -> Mux1/1
  Demux1/3 -> Mux1/3
  Constant/1 -> Mux/2
  Demux/2 -> Terminator/1
  Demux/1 -> Mux/1
  Demux/3 -> Mux/3

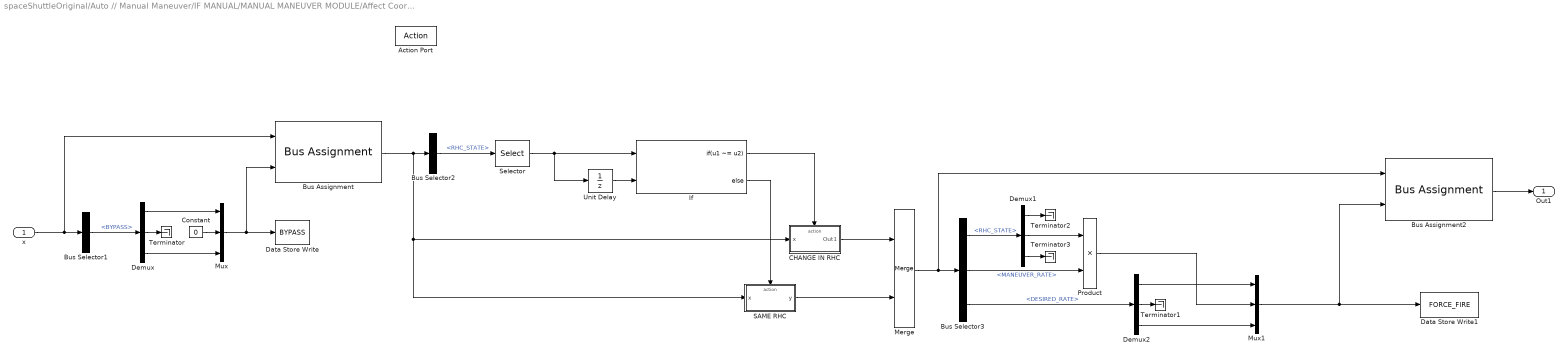
== system spaceShuttleOriginal/Auto // Manual Maneuver/IF MANUAL/MANUAL MANEUVER MODULE/Affect Coordinate 2/CLOSED LOOP = ON ==
  x : Inport
  Action Port : ActionPort  ActionType=then
  Bus Assignment : BusAssignment  AssignedSignals=BYPASS
  Bus Assignment2 : BusAssignment  AssignedSignals=FORCE_FIRE
  Bus Selector1 : BusSelector  OutputSignals=BYPASS
  Bus Selector2 : BusSelector  OutputSignals=USER_INPUTS.RHC_STATE
  Bus Selector3 : BusSelector  OutputSignals=USER_INPUTS.RHC_STATE,USER_INPUTS.MANEUVER_RATE,DESIRED_RATE
  CHANGE IN RHC : Subsystem  TreatAsAtomicUnit=on
  Constant : Constant  Value=0
  Data Store Write : DataStoreWrite  DataStoreName=BYPASS
  Data Store Write1 : DataStoreWrite  DataStoreName=FORCE_FIRE
  Demux : Demux  Outputs=3
  Demux1 : Demux  Outputs=3
  Demux2 : Demux  Outputs=3
  If : If  NumInputs=2  IfExpression=u1 ~= u2
  Merge : Merge
  Mux : Mux  Inputs=3
  Mux1 : Mux  Inputs=3
  Product : Product
  SAME RHC : Subsystem  TreatAsAtomicUnit=on
  Selector : Selector  InputPortWidth=3  IndexOptions=Index vector (dialog)  Indices=[2]  OutputSizes=1
  Terminator{,1..3} (4 alike) : Terminator
  Unit Delay : UnitDelay  SampleTime=-1
  Out1 : Outport
  wires:
  x/1 -> Bus Assignment/1, Bus Selector1/1
  Bus Selector1/1 -> Demux/1  "<BYPASS>"
  Demux/3 -> Mux/3
  Mux/1 -> Data Store Write/1, Bus Assignment/2
  Bus Assignment/1 -> CHANGE IN RHC/1(x), SAME RHC/1(x), Bus Selector2/1
  Bus Selector2/1 -> Selector/1  "<RHC_STATE>"
  Selector/1 -> Unit Delay/1, If/1
  Unit Delay/1 -> If/2
  SAME RHC/1(y) -> Merge/2
  If/2 -> SAME RHC/Action
  If/1 -> CHANGE IN RHC/Action
  CHANGE IN RHC/1(Out1) -> Merge/1
  Constant/1 -> Mux/2
  Demux/1 -> Mux/1
  Mux1/1 -> Bus Assignment2/2, Data Store Write1/1
  Demux2/3 -> Mux1/3
  Bus Selector3/2 -> Product/2  "<MANEUVER_RATE>"
  Bus Selector3/1 -> Demux1/1  "<RHC_STATE>"
  Bus Selector3/3 -> Demux2/1  "<DESIRED_RATE>"
  Bus Assignment2/1 -> Out1/1
  Merge/1 -> Bus Assignment2/1, Bus Selector3/1
  Demux1/2 -> Product/1
  Product/1 -> Mux1/2
  Demux2/1 -> Mux1/1
  Demux/2 -> Terminator/1
  Demux2/2 -> Terminator1/1
  Demux1/1 -> Terminator2/1
  Demux1/3 -> Terminator3/1

== system spaceShuttleOriginal/Auto // Manual Maneuver/IF MANUAL/MANUAL MANEUVER MODULE/Affect Coordinate 3/CLOSED LOOP = OFF ==
  x : Inport
  Action Port : ActionPort  ActionType=else
  Bus Assignment : BusAssignment  AssignedSignals=BYPASS
  Bus Assignment1 : BusAssignment  AssignedSignals=ROTATION_COMMAND
  Bus Selector : BusSelector  OutputSignals=BYPASS
  Bus Selector1 : BusSelector  OutputSignals=USER_INPUTS.RHC_STATE
  Bus Selector2 : BusSelector  OutputSignals=ROTATION_COMMAND
  Constant : Constant
  Data Store Write : DataStoreWrite  DataStoreName=BYPASS
  Data Store Write1 : DataStoreWrite  DataStoreName=ROTATION_COMMAND
  Demux : Demux  Outputs=3
  Demux1 : Demux  Outputs=3
  Mux : Mux  Inputs=3
  Mux1 : Mux  Inputs=3
  Selector : Selector  InputPortWidth=3  IndexOptions=Index vector (dialog)  Indices=[3]  OutputSizes=1
  Terminator : Terminator
  Terminator1 : Terminator
  y : Outport
  wires:
  x/1 -> Bus Assignment/1, Bus Selector/1
  Bus Selector/1 -> Demux/1  "<BYPASS>"
  Mux/1 -> Data Store Write/1, Bus Assignment/2
  Demux/1 -> Mux/1
  Bus Assignment/1 -> Bus Assignment1/1, Bus Selector1/1, Bus Selector2/1
  Mux1/1 -> Data Store Write1/1, Bus Assignment1/2
  Bus Selector2/1 -> Demux1/1  "<ROTATION_COMMAND>"
  Bus Selector1/1 -> Selector/1  "<RHC_STATE>"
  Bus Assignment1/1 -> y/1
  Constant/1 -> Mux/3
  Demux/3 -> Terminator/1
  Demux/2 -> Mux/2
  Demux1/3 -> Terminator1/1
  Demux1/1 -> Mux1/1
  Demux1/2 -> Mux1/2
  Selector/1 -> Mux1/3

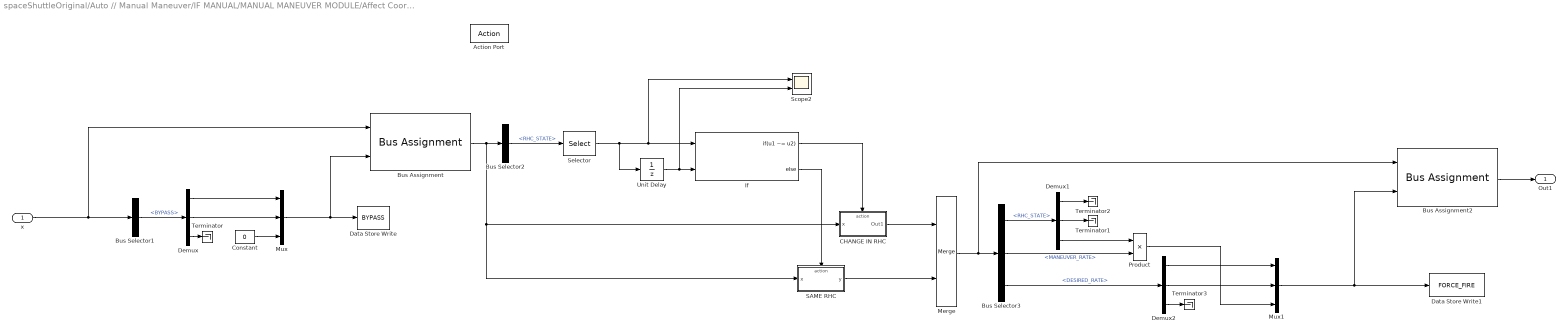
== system spaceShuttleOriginal/Auto // Manual Maneuver/IF MANUAL/MANUAL MANEUVER MODULE/Affect Coordinate 3/CLOSED LOOP = ON ==
  x : Inport
  Action Port : ActionPort  ActionType=then
  Bus Assignment : BusAssignment  AssignedSignals=BYPASS
  Bus Assignment2 : BusAssignment  AssignedSignals=FORCE_FIRE
  Bus Selector1 : BusSelector  OutputSignals=BYPASS
  Bus Selector2 : BusSelector  OutputSignals=USER_INPUTS.RHC_STATE
  Bus Selector3 : BusSelector  OutputSignals=USER_INPUTS.RHC_STATE,USER_INPUTS.MANEUVER_RATE,DESIRED_RATE
  CHANGE IN RHC : Subsystem  TreatAsAtomicUnit=on
  Constant : Constant  Value=0
  Data Store Write : DataStoreWrite  DataStoreName=BYPASS
  Data Store Write1 : DataStoreWrite  DataStoreName=FORCE_FIRE
  Demux : Demux  Outputs=3
  Demux1 : Demux  Outputs=3
  Demux2 : Demux  Outputs=3
  If : If  NumInputs=2  IfExpression=u1 ~= u2
  Merge : Merge
  Mux : Mux  Inputs=3
  Mux1 : Mux  Inputs=3
  Product : Product
  SAME RHC : Subsystem  TreatAsAtomicUnit=on
  Scope2 : Scope  NumInputPorts=2
  Selector : Selector  InputPortWidth=3  IndexOptions=Index vector (dialog)  Indices=[3]  OutputSizes=1
  Terminator{,1..3} (4 alike) : Terminator
  Unit Delay : UnitDelay  SampleTime=-1
  Out1 : Outport
  wires:
  x/1 -> Bus Assignment/1, Bus Selector1/1
  Bus Selector1/1 -> Demux/1  "<BYPASS>"
  Mux/1 -> Data Store Write/1, Bus Assignment/2
  Bus Assignment/1 -> CHANGE IN RHC/1(x), SAME RHC/1(x), Bus Selector2/1
  Bus Selector2/1 -> Selector/1  "<RHC_STATE>"
  Selector/1 -> Unit Delay/1, Scope2/1, If/1
  Unit Delay/1 -> Scope2/2, If/2
  SAME RHC/1(y) -> Merge/2
  If/2 -> SAME RHC/Action
  If/1 -> CHANGE IN RHC/Action
  CHANGE IN RHC/1(Out1) -> Merge/1
  Constant/1 -> Mux/3
  Demux/2 -> Mux/2
  Demux/1 -> Mux/1
  Bus Selector3/3 -> Demux2/1  "<DESIRED_RATE>"
  Bus Assignment2/1 -> Out1/1
  Bus Selector3/2 -> Product/2  "<MANEUVER_RATE>"
  Bus Selector3/1 -> Demux1/1  "<RHC_STATE>"
  Merge/1 -> Bus Assignment2/1, Bus Selector3/1
  Mux1/1 -> Bus Assignment2/2, Data Store Write1/1
  Demux1/3 -> Product/1
  Product/1 -> Mux1/3
  Demux2/1 -> Mux1/1
  Demux2/2 -> Mux1/2
  Demux/3 -> Terminator/1
  Demux1/2 -> Terminator1/1
  Demux1/1 -> Terminator2/1
  Demux2/3 -> Terminator3/1

== system spaceShuttleOriginal/Auto // Manual Maneuver/If AUTO/IF COUNTER=0/AUTO MANEUVER MODULE/CHANGE MANEUVER HOLD SW TO OFF ==
  x : Inport
  Action Port : ActionPort  ActionType=elseif
  Bus Assignment : BusAssignment  AssignedSignals=MANEUVER_HOLD_SW
  Constant : Constant  Value=0
  Data Store Read : DataStoreRead  DataStoreName=MANEUVER_HOLD_SW  DataStoreElements=MANEUVER_HOLD_SW(1)
  Data Store Write : DataStoreWrite  DataStoreName=MANEUVER_HOLD_SW
  Mux : Mux  Inputs=2
  Out1 : Outport
  wires:
  x/1 -> Bus Assignment/1
  Constant/1 -> Mux/1
  Mux/1 -> Bus Assignment/2, Data Store Write/1
  Bus Assignment/1 -> Out1/1
  Data Store Read/1 -> Mux/2

== system spaceShuttleOriginal/Auto // Manual Maneuver/If AUTO/IF COUNTER=0/AUTO MANEUVER MODULE/CHANGE MANEUVER HOLD SW TO ON ==
  x : Inport
  Action Port : ActionPort  ActionType=then
  Bus Assignment : BusAssignment  AssignedSignals=MANEUVER_HOLD_SW
  Constant : Constant
  Data Store Read : DataStoreRead  DataStoreName=MANEUVER_HOLD_SW  DataStoreElements=MANEUVER_HOLD_SW(1)
  Data Store Write : DataStoreWrite  DataStoreName=MANEUVER_HOLD_SW
  Mux : Mux  Inputs=2
  Out1 : Outport
  wires:
  x/1 -> Bus Assignment/1
  Bus Assignment/1 -> Out1/1
  Constant/1 -> Mux/1
  Data Store Read/1 -> Mux/2
  Mux/1 -> Bus Assignment/2, Data Store Write/1

== system spaceShuttleOriginal/Auto // Manual Maneuver/If AUTO/IF COUNTER=0/AUTO MANEUVER MODULE/GET CONTROL ACCELERATION ==
  PRIMARY VERNIER SW : Inport
  If : If  IfExpression=u1 == 1
  Merge : Merge
  PRIMARY : Subsystem  TreatAsAtomicUnit=on
  VERNIER : Subsystem  TreatAsAtomicUnit=on
  CA : Outport
  wires:
  If/2 -> VERNIER/Action
  If/1 -> PRIMARY/Action
  PRIMARY VERNIER SW/1 -> If/1
  PRIMARY/1(Out1) -> Merge/1
  VERNIER/1(Out2) -> Merge/2
  Merge/1 -> CA/1

== system spaceShuttleOriginal/Auto // Manual Maneuver/If AUTO/IF COUNTER=0/AUTO MANEUVER MODULE/MANEUVER HOLD SW = OFF ==
  x : Inport
  EIGEN AXIS : Inport  Port=2
  ROTATION ANGLE : Inport  Port=3
  Action Port : ActionPort  ActionType=then
  Add : Sum
  Bus Assignment : BusAssignment  AssignedSignals=DESIRED_RATE,DESIRED_ATTITUDE
  Bus Selector2 : BusSelector  OutputSignals=ATTITUDE_ESTIMATE
  Constant : Constant  Value=[0;0;0]
  Data Store Write : DataStoreWrite  DataStoreName=DESIRED_RATE
  Data Store Write1 : DataStoreWrite  DataStoreName=DESIRED_ATTITUDE
  Product : Product
  Out1 : Outport
  wires:
  x/1 -> Bus Assignment/1, Bus Selector2/1
  Bus Assignment/1 -> Out1/1
  Constant/1 -> Bus Assignment/2, Data Store Write/1
  Add/1 -> Bus Assignment/3, Data Store Write1/1
  ROTATION ANGLE/1 -> Product/2
  Bus Selector2/1 -> Add/1  "<ATTITUDE_ESTIMATE>"
  EIGEN AXIS/1 -> Product/1
  Product/1 -> Add/2

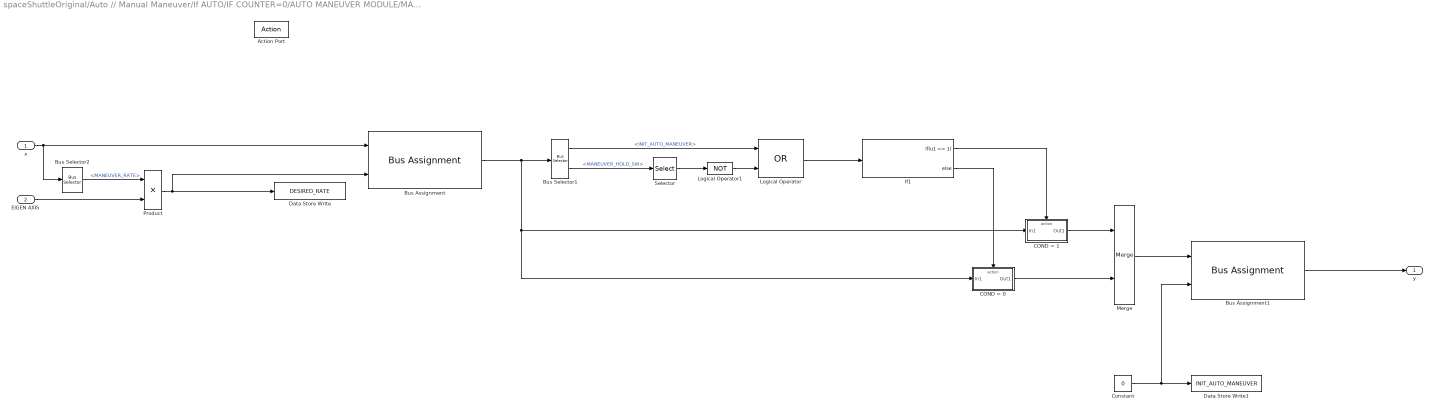
== system spaceShuttleOriginal/Auto // Manual Maneuver/If AUTO/IF COUNTER=0/AUTO MANEUVER MODULE/MANEUVER HOLD SW = ON ==
  x : Inport
  EIGEN AXIS : Inport  Port=2
  Action Port : ActionPort  ActionType=else
  Bus Assignment : BusAssignment  AssignedSignals=DESIRED_RATE
  Bus Assignment1 : BusAssignment  AssignedSignals=INIT_AUTO_MANEUVER
  Bus Selector1 : BusSelector  OutputSignals=INIT_AUTO_MANEUVER,MANEUVER_HOLD_SW
  Bus Selector2 : BusSelector  OutputSignals=USER_INPUTS.MANEUVER_RATE
  COND = 0 : Subsystem  TreatAsAtomicUnit=on
  COND = 1 : Subsystem  TreatAsAtomicUnit=on
  Constant : Constant  Value=0
  Data Store Write : DataStoreWrite  DataStoreName=DESIRED_RATE
  Data Store Write1 : DataStoreWrite  DataStoreName=INIT_AUTO_MANEUVER
  If1 : If  IfExpression=u1 == 1
  Logical Operator : Logic  Operator=OR  AllPortsSameDT=off  OutDataTypeStr=boolean
  Logical Operator1 : Logic  Operator=NOT  AllPortsSameDT=off  OutDataTypeStr=boolean
  Merge : Merge
  Product : Product
  Selector : Selector  InputPortWidth=2  IndexOptions=Index vector (dialog)  Indices=[2]  OutputSizes=1
  y : Outport
  wires:
  x/1 -> Bus Assignment/1, Bus Selector2/1
  Bus Selector2/1 -> Product/1  "<MANEUVER_RATE>"
  EIGEN AXIS/1 -> Product/2
  Product/1 -> Data Store Write/1, Bus Assignment/2
  Selector/1 -> Logical Operator1/1
  Bus Selector1/2 -> Selector/1  "<MANEUVER_HOLD_SW>"
  Bus Selector1/1 -> Logical Operator/1  "<INIT_AUTO_MANEUVER>"
  Logical Operator1/1 -> Logical Operator/2
  Logical Operator/1 -> If1/1
  If1/2 -> COND = 0/Action
  COND = 0/1(Out1) -> Merge/2
  Bus Assignment/1 -> COND = 1/1(In1), COND = 0/1(In1), Bus Selector1/1
  If1/1 -> COND = 1/Action
  COND = 1/1(Out1) -> Merge/1
  Merge/1 -> Bus Assignment1/1
  Bus Assignment1/1 -> y/1
  Constant/1 -> Bus Assignment1/2, Data Store Write1/1

== system spaceShuttleOriginal/Auto // Manual Maneuver/IF MANUAL/MANUAL MANEUVER MODULE/Affect Coordinate 1/CLOSED LOOP = ON/CHANGE IN RHC ==
  x : Inport
  Action Port : ActionPort  ActionType=then
  Bus Assignment : BusAssignment  AssignedSignals=BYPASS
  Bus Selector1 : BusSelector  OutputSignals=INIT_STATE_ERROR
  Bus Selector2 : BusSelector  OutputSignals=USER_INPUTS.RHC_STATE
  Constant : Constant
  Data Store Write : DataStoreWrite  DataStoreName=INIT_STATE_ERROR
  Demux : Demux  Outputs=3
  If : If  IfExpression=u1 ~= 0
  Merge : Merge
  Mux : Mux  Inputs=3
  RHC 0 : Subsystem  TreatAsAtomicUnit=on
  RHC NOT 0 : Subsystem  TreatAsAtomicUnit=on
  Selector : Selector  InputPortWidth=3  IndexOptions=Index vector (dialog)  Indices=[1]  OutputSizes=1
  Terminator : Terminator
  Out1 : Outport
  wires:
  Mux/1 -> Data Store Write/1, Bus Assignment/2
  Bus Selector1/1 -> Demux/1  "<INIT_STATE_ERROR>"
  x/1 -> Bus Assignment/1, Bus Selector1/1
  Constant/1 -> Mux/1
  Demux/2 -> Mux/2
  Demux/3 -> Mux/3
  If/2 -> RHC 0/Action
  RHC 0/1(y) -> Merge/2
  If/1 -> RHC NOT 0/Action
  RHC NOT 0/1(y) -> Merge/1
  Bus Assignment/1 -> RHC 0/1(x), RHC NOT 0/1(x), Bus Selector2/1
  Bus Selector2/1 -> Selector/1  "<RHC_STATE>"
  Selector/1 -> If/1
  Merge/1 -> Out1/1
  Demux/1 -> Terminator/1

== system spaceShuttleOriginal/Auto // Manual Maneuver/IF MANUAL/MANUAL MANEUVER MODULE/Affect Coordinate 1/CLOSED LOOP = ON/SAME RHC ==
  x : Inport
  Action Port : ActionPort  ActionType=else
  y : Outport
  wires:
  x/1 -> y/1

== system spaceShuttleOriginal/Auto // Manual Maneuver/IF MANUAL/MANUAL MANEUVER MODULE/Affect Coordinate 2/CLOSED LOOP = ON/CHANGE IN RHC ==
  x : Inport
  Action Port : ActionPort  ActionType=then
  Bus Assignment : BusAssignment  AssignedSignals=BYPASS
  Bus Selector1 : BusSelector  OutputSignals=INIT_STATE_ERROR
  Bus Selector2 : BusSelector  OutputSignals=USER_INPUTS.RHC_STATE
  Constant : Constant
  Data Store Write : DataStoreWrite  DataStoreName=INIT_STATE_ERROR
  Demux : Demux  Outputs=3
  If : If  IfExpression=u1 ~= 0
  Merge : Merge
  Mux : Mux  Inputs=3
  RHC 0 : Subsystem  TreatAsAtomicUnit=on
  RHC NOT 0 : Subsystem  TreatAsAtomicUnit=on
  Selector : Selector  InputPortWidth=3  IndexOptions=Index vector (dialog)  Indices=[2]  OutputSizes=1
  Terminator : Terminator
  Out1 : Outport
  wires:
  Mux/1 -> Data Store Write/1, Bus Assignment/2
  Bus Selector1/1 -> Demux/1  "<INIT_STATE_ERROR>"
  x/1 -> Bus Assignment/1, Bus Selector1/1
  If/2 -> RHC 0/Action
  RHC 0/1(y) -> Merge/2
  If/1 -> RHC NOT 0/Action
  RHC NOT 0/1(y) -> Merge/1
  Bus Assignment/1 -> RHC 0/1(x), RHC NOT 0/1(x), Bus Selector2/1
  Bus Selector2/1 -> Selector/1  "<RHC_STATE>"
  Selector/1 -> If/1
  Constant/1 -> Mux/2
  Demux/3 -> Mux/3
  Demux/1 -> Mux/1
  Merge/1 -> Out1/1
  Demux/2 -> Terminator/1

== system spaceShuttleOriginal/Auto // Manual Maneuver/IF MANUAL/MANUAL MANEUVER MODULE/Affect Coordinate 2/CLOSED LOOP = ON/SAME RHC ==
  x : Inport
  Action Port : ActionPort  ActionType=else
  y : Outport
  wires:
  x/1 -> y/1

== system spaceShuttleOriginal/Auto // Manual Maneuver/IF MANUAL/MANUAL MANEUVER MODULE/Affect Coordinate 3/CLOSED LOOP = ON/CHANGE IN RHC ==
  x : Inport
  Action Port : ActionPort  ActionType=then
  Bus Assignment : BusAssignment  AssignedSignals=BYPASS
  Bus Selector1 : BusSelector  OutputSignals=INIT_STATE_ERROR
  Bus Selector2 : BusSelector  OutputSignals=USER_INPUTS.RHC_STATE
  Constant : Constant
  Data Store Write : DataStoreWrite  DataStoreName=INIT_STATE_ERROR
  Demux : Demux  Outputs=3
  If : If  IfExpression=u1 ~= 0
  Merge : Merge
  Mux : Mux  Inputs=3
  RHC 0 : Subsystem  TreatAsAtomicUnit=on
  RHC NOT 0 : Subsystem  TreatAsAtomicUnit=on
  Selector : Selector  InputPortWidth=3  IndexOptions=Index vector (dialog)  Indices=[3]  OutputSizes=1
  Terminator : Terminator
  Out1 : Outport
  wires:
  Mux/1 -> Data Store Write/1, Bus Assignment/2
  Bus Selector1/1 -> Demux/1  "<INIT_STATE_ERROR>"
  x/1 -> Bus Assignment/1, Bus Selector1/1
  If/2 -> RHC 0/Action
  RHC 0/1(y) -> Merge/2
  If/1 -> RHC NOT 0/Action
  RHC NOT 0/1(y) -> Merge/1
  Bus Assignment/1 -> RHC 0/1(x), RHC NOT 0/1(x), Bus Selector2/1
  Bus Selector2/1 -> Selector/1  "<RHC_STATE>"
  Selector/1 -> If/1
  Constant/1 -> Mux/3
  Demux/2 -> Mux/2
  Demux/1 -> Mux/1
  Merge/1 -> Out1/1
  Demux/3 -> Terminator/1

== system spaceShuttleOriginal/Auto // Manual Maneuver/IF MANUAL/MANUAL MANEUVER MODULE/Affect Coordinate 3/CLOSED LOOP = ON/SAME RHC ==
  x : Inport
  Action Port : ActionPort  ActionType=else
  y : Outport
  wires:
  x/1 -> y/1

== system spaceShuttleOriginal/Auto // Manual Maneuver/If AUTO/IF COUNTER=0/AUTO MANEUVER MODULE/GET CONTROL ACCELERATION/PRIMARY ==
  Action Port : ActionPort  ActionType=then
  Constant1 : Constant  Value=0.8
  Constant3 : Constant  Value=0.9
  Constant4 : Constant  Value=0.6
  Mux : Mux  Inputs=3
  Out1 : Outport
  wires:
  Constant1/1 -> Mux/1
  Constant3/1 -> Mux/2
  Constant4/1 -> Mux/3
  Mux/1 -> Out1/1

== system spaceShuttleOriginal/Auto // Manual Maneuver/If AUTO/IF COUNTER=0/AUTO MANEUVER MODULE/GET CONTROL ACCELERATION/VERNIER ==
  Action Port : ActionPort  ActionType=else
  Constant1 : Constant  Value=0.019
  Constant3 : Constant  Value=0.013
  Constant4 : Constant  Value=0.014
  Mux : Mux  Inputs=3
  Out2 : Outport
  wires:
  Mux/1 -> Out2/1
  Constant4/1 -> Mux/3
  Constant3/1 -> Mux/2
  Constant1/1 -> Mux/1

== system spaceShuttleOriginal/Auto // Manual Maneuver/If AUTO/IF COUNTER=0/AUTO MANEUVER MODULE/MANEUVER HOLD SW = ON/COND = 0 ==
  In1 : Inport
  Action Port : ActionPort  ActionType=else
  Out1 : Outport
  wires:
  In1/1 -> Out1/1

== system spaceShuttleOriginal/Auto // Manual Maneuver/If AUTO/IF COUNTER=0/AUTO MANEUVER MODULE/MANEUVER HOLD SW = ON/COND = 1 ==
  In1 : Inport
  Action Port : ActionPort  ActionType=then
  Add : Sum  Inputs=+-
  Add1 : Sum
  Bus Assignment : BusAssignment  AssignedSignals=DESIRED_ATTITUDE
  Bus Selector1 : BusSelector  OutputSignals=DESIRED_ATTITUDE,RATE_ESTIMATE,USER_INPUTS.PRIMARY_VERNIER_SW,ATTITUDE_ESTIMATE
  Data Store Write : DataStoreWrite  DataStoreName=DESIRED_ATTITUDE
  Demux : Demux  Outputs=3
  Demux1 : Demux  Outputs=3
  Divide : Product  Inputs=*/
  Divide1 : Product  Inputs=*/
  Divide2 : Product  Inputs=*/
  GET CONTROL ACCELERATION : Subsystem
  Mux : Mux  Inputs=3
  Sub Sysyem1 : Subsystem
  Sub Sysyem2 : Subsystem
  Sub Sysyem3 : Subsystem
  Out1 : Outport
  wires:
  In1/1 -> Bus Assignment/1, Bus Selector1/1
  Bus Selector1/1 -> Add/1  "<DESIRED_ATTITUDE>"
  Bus Selector1/2 -> Add/2  "<RATE_ESTIMATE>"
  Add/1 -> Demux/1
  Bus Selector1/3 -> GET CONTROL ACCELERATION/1(PRIMARY VERNIER SW)  "<PRIMARY_VERNIER_SW>"
  GET CONTROL ACCELERATION/1(CA) -> Demux1/1
  Demux/1 -> Sub Sysyem1/1(In1)
  Demux/2 -> Sub Sysyem2/1(In1)
  Demux/3 -> Sub Sysyem3/1(In1)
  Sub Sysyem1/1(Out1) -> Divide/1
  Demux1/1 -> Divide/2
  Sub Sysyem2/1(Out1) -> Divide1/1
  Demux1/2 -> Divide1/2
  Sub Sysyem3/1(Out1) -> Divide2/1
  Demux1/3 -> Divide2/2
  Divide/1 -> Mux/1
  Divide1/1 -> Mux/2
  Divide2/1 -> Mux/3
  Mux/1 -> Add1/1
  Bus Selector1/4 -> Add1/2  "<ATTITUDE_ESTIMATE>"
  Bus Assignment/1 -> Out1/1
  Add1/1 -> Data Store Write/1, Bus Assignment/2

== system spaceShuttleOriginal/Auto // Manual Maneuver/IF MANUAL/MANUAL MANEUVER MODULE/Affect Coordinate 1/CLOSED LOOP = ON/CHANGE IN RHC/RHC 0 ==
  x : Inport
  Action Port : ActionPort  ActionType=else
  y : Outport
  wires:
  x/1 -> y/1

== system spaceShuttleOriginal/Auto // Manual Maneuver/IF MANUAL/MANUAL MANEUVER MODULE/Affect Coordinate 1/CLOSED LOOP = ON/CHANGE IN RHC/RHC NOT 0 ==
  x : Inport
  Action Port : ActionPort  ActionType=then
  Bus Assignment : BusAssignment  AssignedSignals=FORCE_FIRE
  Bus Selector1 : BusSelector  OutputSignals=FORCE_FIRE
  Constant : Constant
  Data Store Write : DataStoreWrite  DataStoreName=FORCE_FIRE
  Demux : Demux  Outputs=3
  Mux : Mux  Inputs=3
  Terminator : Terminator
  y : Outport
  wires:
  Mux/1 -> Data Store Write/1, Bus Assignment/2
  Bus Selector1/1 -> Demux/1  "<FORCE_FIRE>"
  x/1 -> Bus Assignment/1, Bus Selector1/1
  Constant/1 -> Mux/1
  Demux/2 -> Mux/2
  Demux/3 -> Mux/3
  Bus Assignment/1 -> y/1
  Demux/1 -> Terminator/1

== system spaceShuttleOriginal/Auto // Manual Maneuver/IF MANUAL/MANUAL MANEUVER MODULE/Affect Coordinate 2/CLOSED LOOP = ON/CHANGE IN RHC/RHC 0 ==
  x : Inport
  Action Port : ActionPort  ActionType=else
  y : Outport
  wires:
  x/1 -> y/1

== system spaceShuttleOriginal/Auto // Manual Maneuver/IF MANUAL/MANUAL MANEUVER MODULE/Affect Coordinate 2/CLOSED LOOP = ON/CHANGE IN RHC/RHC NOT 0 ==
  x : Inport
  Action Port : ActionPort  ActionType=then
  Bus Assignment : BusAssignment  AssignedSignals=FORCE_FIRE
  Bus Selector1 : BusSelector  OutputSignals=FORCE_FIRE
  Constant : Constant
  Data Store Write : DataStoreWrite  DataStoreName=FORCE_FIRE
  Demux : Demux  Outputs=3
  Mux : Mux  Inputs=3
  Terminator : Terminator
  y : Outport
  wires:
  Mux/1 -> Data Store Write/1, Bus Assignment/2
  Bus Selector1/1 -> Demux/1  "<FORCE_FIRE>"
  x/1 -> Bus Assignment/1, Bus Selector1/1
  Bus Assignment/1 -> y/1
  Constant/1 -> Mux/2
  Demux/3 -> Mux/3
  Demux/1 -> Mux/1
  Demux/2 -> Terminator/1

== system spaceShuttleOriginal/Auto // Manual Maneuver/IF MANUAL/MANUAL MANEUVER MODULE/Affect Coordinate 3/CLOSED LOOP = ON/CHANGE IN RHC/RHC 0 ==
  x : Inport
  Action Port : ActionPort  ActionType=else
  y : Outport
  wires:
  x/1 -> y/1

== system spaceShuttleOriginal/Auto // Manual Maneuver/IF MANUAL/MANUAL MANEUVER MODULE/Affect Coordinate 3/CLOSED LOOP = ON/CHANGE IN RHC/RHC NOT 0 ==
  x : Inport
  Action Port : ActionPort  ActionType=then
  Bus Assignment : BusAssignment  AssignedSignals=FORCE_FIRE
  Bus Selector1 : BusSelector  OutputSignals=FORCE_FIRE
  Constant : Constant
  Data Store Write : DataStoreWrite  DataStoreName=FORCE_FIRE
  Demux : Demux  Outputs=3
  Mux : Mux  Inputs=3
  Terminator : Terminator
  y : Outport
  wires:
  Mux/1 -> Data Store Write/1, Bus Assignment/2
  Bus Selector1/1 -> Demux/1  "<FORCE_FIRE>"
  x/1 -> Bus Assignment/1, Bus Selector1/1
  Bus Assignment/1 -> y/1
  Constant/1 -> Mux/3
  Demux/2 -> Mux/2
  Demux/1 -> Mux/1
  Demux/3 -> Terminator/1

== system spaceShuttleOriginal/Auto // Manual Maneuver/If AUTO/IF COUNTER=0/AUTO MANEUVER MODULE/MANEUVER HOLD SW = ON/COND = 1/GET CONTROL ACCELERATION ==
  PRIMARY VERNIER SW : Inport
  If : If  IfExpression=u1 == 1
  Merge : Merge
  PRIMARY : Subsystem  TreatAsAtomicUnit=on
  VERNIER : Subsystem  TreatAsAtomicUnit=on
  CA : Outport
  wires:
  If/2 -> VERNIER/Action
  If/1 -> PRIMARY/Action
  PRIMARY VERNIER SW/1 -> If/1
  PRIMARY/1(Out1) -> Merge/1
  VERNIER/1(Out2) -> Merge/2
  Merge/1 -> CA/1

== system spaceShuttleOriginal/Auto // Manual Maneuver/If AUTO/IF COUNTER=0/AUTO MANEUVER MODULE/MANEUVER HOLD SW = ON/COND = 1/Sub Sysyem1 ==
  In1 : Inport
  Abs : Abs
  Gain : Gain  Gain=-1
  Product : Product
  Out1 : Outport
  wires:
  Product/1 -> Gain/1
  In1/1 -> Product/1, Abs/1
  Abs/1 -> Product/2
  Gain/1 -> Out1/1

== system spaceShuttleOriginal/Auto // Manual Maneuver/If AUTO/IF COUNTER=0/AUTO MANEUVER MODULE/MANEUVER HOLD SW = ON/COND = 1/Sub Sysyem2 ==
  In1 : Inport
  Abs : Abs
  Gain : Gain  Gain=-1
  Product : Product
  Out1 : Outport
  wires:
  Product/1 -> Gain/1
  In1/1 -> Product/1, Abs/1
  Abs/1 -> Product/2
  Gain/1 -> Out1/1

== system spaceShuttleOriginal/Auto // Manual Maneuver/If AUTO/IF COUNTER=0/AUTO MANEUVER MODULE/MANEUVER HOLD SW = ON/COND = 1/Sub Sysyem3 ==
  In1 : Inport
  Abs : Abs
  Gain : Gain  Gain=-1
  Product : Product
  Out1 : Outport
  wires:
  Product/1 -> Gain/1
  In1/1 -> Product/1, Abs/1
  Abs/1 -> Product/2
  Gain/1 -> Out1/1

== system spaceShuttleOriginal/Auto // Manual Maneuver/If AUTO/IF COUNTER=0/AUTO MANEUVER MODULE/MANEUVER HOLD SW = ON/COND = 1/GET CONTROL ACCELERATION/PRIMARY ==
  Action Port : ActionPort  ActionType=then
  Constant1 : Constant  Value=0.8
  Constant3 : Constant  Value=0.9
  Constant4 : Constant  Value=0.6
  Mux : Mux  Inputs=3
  Out1 : Outport
  wires:
  Constant1/1 -> Mux/1
  Constant3/1 -> Mux/2
  Constant4/1 -> Mux/3
  Mux/1 -> Out1/1

== system spaceShuttleOriginal/Auto // Manual Maneuver/If AUTO/IF COUNTER=0/AUTO MANEUVER MODULE/MANEUVER HOLD SW = ON/COND = 1/GET CONTROL ACCELERATION/VERNIER ==
  Action Port : ActionPort  ActionType=else
  Constant1 : Constant  Value=0.019
  Constant3 : Constant  Value=0.013
  Constant4 : Constant  Value=0.014
  Mux : Mux  Inputs=3
  Out2 : Outport
  wires:
  Mux/1 -> Out2/1
  Constant4/1 -> Mux/3
  Constant3/1 -> Mux/2
  Constant1/1 -> Mux/1
